simulink subsystem "robot"  (R2023a)
settings: Solver=VariableStepAuto  StartTime=0.0  StopTime=10.0  RelTol=1e-3
model mask{K=7, T1=0.1, T2=0.05, ki=0, kp=0, kd=0}
  mask prompts: K "Коэффициент усиления"; T1 "(Частота перекючения 1)^-1"; T2 "(Частота перекючения 2)^-1"; ki "коэффициент интегральной связи"; kp "коэффициент прямой связи"; kd "коэффициент дифференциальной связи"
settings Model: Creator=diontep  LastModifiedBy=diontep

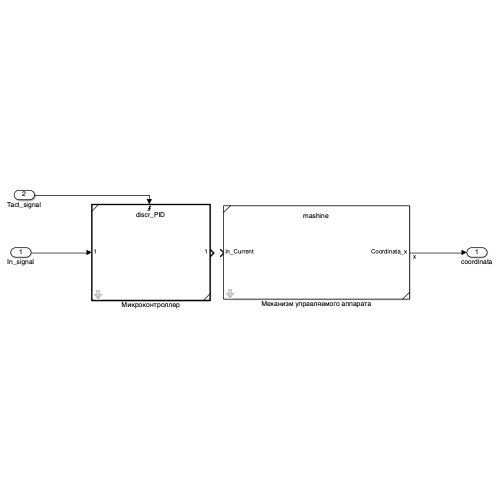
[thumbnail: Simulink's stored preview of the top-level diagram]
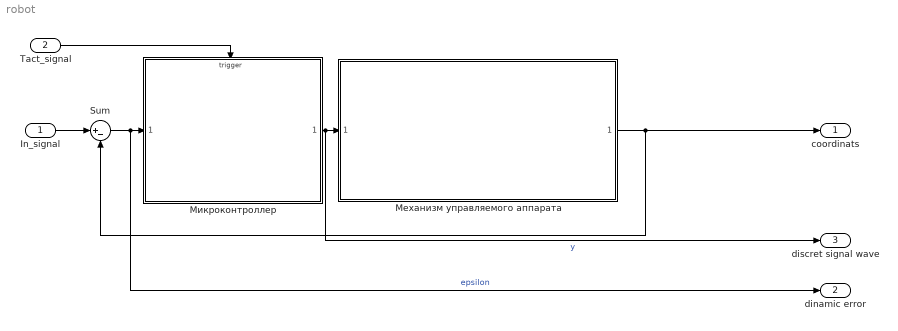
== system robot ==
  In_signal : Inport
  Tact_signal : Inport  Port=2
  Sum : Sum  Inputs=|+-
  Механизм управляемого аппарата : Subsystem  ReferencedSubsystem=mashine  k=K  T1=T1  T2=T2
  Микроконтроллер : Subsystem  ReferencedSubsystem=discr_PID  ki=ki  kp=kp  kd=kd
  coordinats : Outport
  dinamic error : Outport  Port=2
  discret signal wave : Outport  Port=3
  wires:
  In_signal/1 -> Sum/1
  Tact_signal/1 -> Микроконтроллер/Trigger
  Механизм управляемого аппарата/1 -> Sum/2, coordinats/1
  Sum/1 -> Микроконтроллер/1, dinamic error/1  "epsilon"
  Микроконтроллер/1 -> Механизм управляемого аппарата/1, discret signal wave/1  "y"
